simulink model "Local_trajectory_generate"  (R2021a)
settings: configuration reference "AION_IDS_Speedgoat" (kept outside this file)
undefined symbols (not defined in the file): MAX_GLOBAL_TRAJECTORY_WAY_POINT_NUMBER, ReferenceTrajectories
libraries: simulink x1
settings Model: DataDictionary=Local_Trajectory_Generate.sldd  Creator=xinrui  LastModifiedBy=Administrator
settings ConfigSetRef: SourceName=AION_IDS_Speedgoat

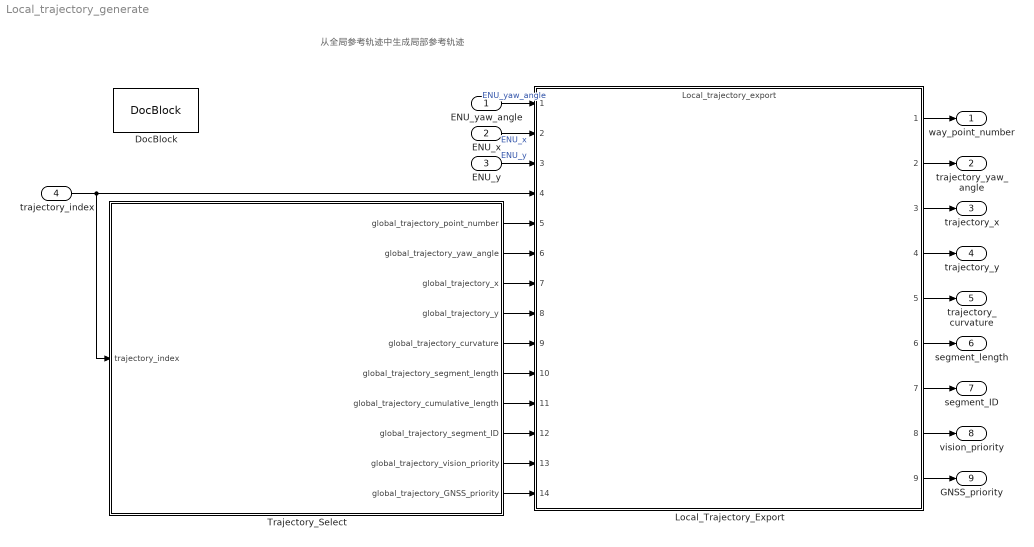
== system Local_trajectory_generate ==
  note: 从全局参考轨迹中生成局部参考轨迹
  ENU_yaw_angle : Inport  OutDataTypeStr=double  PortDimensions=1
  ENU_x : Inport  Port=2  OutDataTypeStr=double  PortDimensions=1
  ENU_y : Inport  Port=3  OutDataTypeStr=double  PortDimensions=1
  trajectory_index : Inport  Port=4  OutDataTypeStr=int8  PortDimensions=1
  DocBlock : simulink/Model-Wide Utilities/DocBlock  DocumentType=HTML  mask(DocBlock){}
      mask Display:
      | plot([.8 0 0 1 1 .8 .8 1],[1 1 0 0 .8 1 .8 .8]);
      | text(.5,.6,'CHANGELOG','horizontalalignment','center');
      | text(.95,.05,get_param(gcb,'DocumentType'),'verticalalignment','bottom','horizontalalignment','right');
  Local_Trajectory_Export : ModelReference  ModelNameDialog=Local_trajectory_export  SimulationMode=Normal  ModelReferenceVersion=4.174
  Trajectory_Select : MATLAB Function  TreatAsAtomicUnit=on
  way_point_number : Outport  OutDataTypeStr=int32  PortDimensions=1
  trajectory_yaw_angle : Outport  Port=2  OutDataTypeStr=double  PortDimensions=MAX_LOCAL_TRAJECTORY_WAY_POINT_NUMBER
  trajectory_x : Outport  Port=3  OutDataTypeStr=double  PortDimensions=MAX_LOCAL_TRAJECTORY_WAY_POINT_NUMBER
  trajectory_y : Outport  Port=4  OutDataTypeStr=double  PortDimensions=MAX_LOCAL_TRAJECTORY_WAY_POINT_NUMBER
  trajectory_curvature : Outport  Port=5  OutDataTypeStr=double  PortDimensions=MAX_LOCAL_TRAJECTORY_WAY_POINT_NUMBER
  segment_length : Outport  Port=6  OutDataTypeStr=double  PortDimensions=MAX_LOCAL_TRAJECTORY_WAY_POINT_NUMBER
  segment_ID : Outport  Port=7  OutDataTypeStr=int8  PortDimensions=MAX_LOCAL_TRAJECTORY_WAY_POINT_NUMBER
  vision_priority : Outport  Port=8  OutDataTypeStr=int8  PortDimensions=MAX_LOCAL_TRAJECTORY_WAY_POINT_NUMBER
  GNSS_priority : Outport  Port=9  OutDataTypeStr=int8  PortDimensions=MAX_LOCAL_TRAJECTORY_WAY_POINT_NUMBER
  wires:
  Trajectory_Select/2(global_trajectory_yaw_angle) -> Local_Trajectory_Export/6
  Local_Trajectory_Export/4 -> trajectory_y/1
  Trajectory_Select/7(global_trajectory_cumulative_length) -> Local_Trajectory_Export/11
  Trajectory_Select/5(global_trajectory_curvature) -> Local_Trajectory_Export/9
  Trajectory_Select/4(global_trajectory_y) -> Local_Trajectory_Export/8
  Trajectory_Select/9(global_trajectory_vision_priority) -> Local_Trajectory_Export/13
  Trajectory_Select/6(global_trajectory_segment_length) -> Local_Trajectory_Export/10
  Local_Trajectory_Export/8 -> vision_priority/1
  Trajectory_Select/3(global_trajectory_x) -> Local_Trajectory_Export/7
  Trajectory_Select/10(global_trajectory_GNSS_priority) -> Local_Trajectory_Export/14
  trajectory_index/1 -> Local_Trajectory_Export/4, Trajectory_Select/1(trajectory_index)
  Trajectory_Select/1(global_trajectory_point_number) -> Local_Trajectory_Export/5
  Trajectory_Select/8(global_trajectory_segment_ID) -> Local_Trajectory_Export/12
  Local_Trajectory_Export/3 -> trajectory_x/1
  Local_Trajectory_Export/5 -> trajectory_curvature/1
  Local_Trajectory_Export/7 -> segment_ID/1
  Local_Trajectory_Export/2 -> trajectory_yaw_angle/1
  Local_Trajectory_Export/6 -> segment_length/1
  ENU_yaw_angle/1 -> Local_Trajectory_Export/1  "ENU_yaw_angle"
  Local_Trajectory_Export/9 -> GNSS_priority/1
  ENU_x/1 -> Local_Trajectory_Export/2  "ENU_x"
  ENU_y/1 -> Local_Trajectory_Export/3  "ENU_y"
  Local_Trajectory_Export/1 -> way_point_number/1

== matlab function Local_trajectory_generate/Trajectory_Select ==
  data: trajectory_index input int8; global_trajectory_point_number output int32; global_trajectory_yaw_angle output double size=MAX_GLOBAL_TRAJECTORY_WAY_POINT_NUMBER; global_trajectory_x output double size=MAX_GLOBAL_TRAJECTORY_WAY_POINT_NUMBER; global_trajectory_y output double size=MAX_GLOBAL_TRAJECTORY_WAY_POINT_NUMBER; global_trajectory_curvature output double size=MAX_GLOBAL_TRAJECTORY_WAY_POINT_NUMBER; global_trajectory_segment_length output double size=MAX_GLOBAL_TRAJECTORY_WAY_POINT_NUMBER; global_trajectory_cumulative_length output double size=MAX_GLOBAL_TRAJECTORY_WAY_POINT_NUMBER; global_trajectory_segment_ID output int8 size=MAX_GLOBAL_TRAJECTORY_WAY_POINT_NUMBER; global_trajectory_vision_priority output int8 size=MAX_GLOBAL_TRAJECTORY_WAY_POINT_NUMBER; global_trajectory_GNSS_priority output int8 size=MAX_GLOBAL_TRAJECTORY_WAY_POINT_NUMBER; ReferenceTrajectories parameter Bus: CONFIG_TRAJECTORIES; MAX_GLOBAL_TRAJECTORY_WAY_POINT_NUMBER parameter double
% 选择参考轨迹
function [global_trajectory_point_number, global_trajectory_yaw_angle, ...
    global_trajectory_x, global_trajectory_y, global_trajectory_curvature, ...
    global_trajectory_segment_length, global_trajectory_cumulative_length, ...
    global_trajectory_segment_ID, global_trajectory_vision_priority, ...
    global_trajectory_GNSS_priority] = Trajectory_select(trajectory_index, ...
    ReferenceTrajectories, MAX_GLOBAL_TRAJECTORY_WAY_POINT_NUMBER)
%   1.输入参数：
%       (1)trajectory_index                          选择的参考轨迹索引，无量纲
%       (2)ReferenceTrajectories                     可供选择的参考轨迹簇，Parameter，保存在数据字典中
%       (3)MAX_GLOBAL_TRAJECTORY_WAY_POINT_NUMBER    全局参考轨迹的最大路点个数，Parameter，保存在数据字典中
%   2.输出参数：
%       (1)global_trajectory_point_number            选择的全局参考轨迹路点数量，无量纲
%       (2)global_trajectory_yaw_angle               选择的全局参考轨迹横摆角数组，deg，有效数据量为global_trajectory_point_number
%       (3)global_trajectory_x                       选择的全局参考轨迹x坐标数组，m，有效数据量为global_trajectory_point_number
%       (4)global_trajectory_y                       选择的全局参考轨迹y坐标数组，m，有效数据量为global_trajectory_point_number
%       (5)global_trajectory_curvature               选择的全局参考轨迹曲率数组，1/m，有效数据量为global_trajectory_point_number
%       (6)global_trajectory_segment_length          选择的全局参考轨迹路点到前一个点的线段长度数组，m，有效数据量为global_trajectory_point_number
%       (7)global_trajectory_cumulative_length       选择的全局参考轨迹路点到起点的累计长度数组，m，有效数据量为global_trajectory_point_number
%       (8)global_trajectory_segment_ID              选择的全局参考轨迹区间代号数组，无量纲，有效数据量为global_trajectory_point_number
%       (9)global_trajectory_vision_priority         选择的全局参考轨迹视觉循迹优先级数组，无量纲，有效数据量为global_trajectory_point_number
%       (10)global_trajectory_GNSS_priority          选择的全局参考轨迹GNSS循迹优先级数组，无量纲，有效数据量为global_trajectory_point_number

%% 静态变量声明及初始化
% 上周期轨迹索引
persistent trajectory_index_previous;
if isempty(trajectory_index_previous)
   trajectory_index_previous = int8(0);
end

%% 输出信号尺寸初始化
global_trajectory_yaw_angle = zeros(MAX_GLOBAL_TRAJECTORY_WAY_POINT_NUMBER, 1);
global_trajectory_x = zeros(MAX_GLOBAL_TRAJECTORY_WAY_POINT_NUMBER, 1);
global_trajectory_y = zeros(MAX_GLOBAL_TRAJECTORY_WAY_POINT_NUMBER, 1);
global_trajectory_curvature = zeros(MAX_GLOBAL_TRAJECTORY_WAY_POINT_NUMBER, 1);
global_trajectory_segment_length = zeros(MAX_GLOBAL_TRAJECTORY_WAY_POINT_NUMBER, 1);
global_trajectory_cumulative_length = zeros(MAX_GLOBAL_TRAJECTORY_WAY_POINT_NUMBER, 1);
global_trajectory_segment_ID = int8(zeros(MAX_GLOBAL_TRAJECTORY_WAY_POINT_NUMBER, 1));
global_trajectory_vision_priority = int8(zeros(MAX_GLOBAL_TRAJECTORY_WAY_POINT_NUMBER, 1));
global_trajectory_GNSS_priority = int8(zeros(MAX_GLOBAL_TRAJECTORY_WAY_POINT_NUMBER, 1));

%% 选择轨迹
% 获取结构体成员名称
namelist = fieldnames(ReferenceTrajectories);

% 初始化
current_trajectory = ReferenceTrajectories.(namelist{1});

% 根据输入索引筛取轨迹
for index = 1 : length(namelist)
    if 1e-4 > abs(trajectory_index - index)
        current_trajectory = ReferenceTrajectories.(namelist{index});
        break;
    end
end

%% 设置输出信号
global_trajectory_point_number = int32(length(current_trajectory.ENU_yaw_angle));
global_trajectory_yaw_angle(1 : global_trajectory_point_number) = ...
    current_trajectory.ENU_yaw_angle;
global_trajectory_x(1 : global_trajectory_point_number) = current_trajectory.ENU_x;
global_trajectory_y(1 : global_trajectory_point_number) = current_trajectory.ENU_y;
global_trajectory_curvature(1 : global_trajectory_point_number) = ...
    current_trajectory.curvature;
global_trajectory_segment_length(1 : global_trajectory_point_number) = ...
    current_trajectory.segment_length;
global_trajectory_cumulative_length(1 : global_trajectory_point_number) = ...
    current_trajectory.cumulative_length;
global_trajectory_segment_ID(1 : global_trajectory_point_number) = ...
    int8(current_trajectory.segment_ID);
global_trajectory_vision_priority(1 : global_trajectory_point_number) = ...
    int8(current_trajectory.vision_priority);
global_trajectory_GNSS_priority(1 : global_trajectory_point_number) = ...
    int8(current_trajectory.GNSS_priority);

%% 相邻周期数据更替
trajectory_index_previous = trajectory_index;

end
